simulink model "sm_tVtest_belt_IdlerArm_i2u0r3_underc"  (R2026a)
settings: Solver=VariableStepAuto  AbsTol=1e-3  EnableMultiTasking=on
undefined symbols (not defined in the file or in its folder): X, Y, Z
libraries: sm_lib x3, nesl_utility x1, sm_trackV_lib_belt_underc_idlerArm_i2u0l3 x1
Description:
  | Undercarriage with Frame and Rollers
  | Copyright 2024-2026 The MathWorks, Inc.
settings Model: Creator=smiller  LastModifiedBy=smiller
settings DebuggingCC: SubsystemReferenceDiagnosticForUnitTest=warning
settings SimscapeCC: SimscapeNominalValues="[{\"value\":\"1\",\"unit\":\"A\"},{\"value\":\"1\",\"unit\":\"bar\"},{\"value\":\"1\",\"unit\":\"cm^2\"},{\"value\":\"1\",\"unit\":\"cm^3/s\"},{\"value\":\"1\",\"unit\":\"kJ/kg\"},{\"value\":\"1\",\"unit\":\"kW\"},{\"value\":\"1\",\"unit\":\"l\"},{\"value\":\"1\",\"unit\":\"N\"},{\"value\":\"1\",\"unit\":\"N*m\"},{\"value\":\"1\",\"unit\":\"V\"}]"  SimscapeLogSimulationStatistics=on
settings DiagnosticsConfigSet: SimMechanicsUnconnectedFramePorts=none
settings ExplorerConfigSet: InternalSimMechanicsExplorerSettings="<ExplorerConfiguration><canonicalview>default</canonicalview><AnimationSetting><BasePlaybackSpeed>1.0</BasePlaybackSpeed><PlaybackSpeedFactor>1.0</PlaybackSpeedFactor></AnimationSetting><TilePanel><TileInfo><Tiles Columns=\"1\" Count=\"1\" Rows=\"1\"><Column Weight=\"1\"/><Row Weight=\"1\"/><Tile Height=\"1\" Width=\"1\" X=\"0\" Y=\"0\"/></Tiles></TileInfo><SceneInfo><SceneViewer><BGColor><R>1</R><G>1</G><B>1</B></BGColor><Camera><DoPerspective>off</DoPerspective><Position><X>0.903819359798529898</X><Y>-1.50805374329867981</Y><Z>-0.0280681494083976357</Z></Position><Center><X>-0.024120903320636794</X><Y>0.0864471732189572295</Y><Z>-0.450624958415139831</Z></Center><Up><X>-0.126434618294550744</X><Y>0.184704601083858</Y><Z>0.974627363475479402</Z></Up><ViewLimDist>1</ViewLimDist><YLim>1.06143678903579719</YLim><XLim>1.81016071934892686</XLim></Camera></SceneViewer></SceneInfo></TilePanel><MechEditorPanel><Cameras/><GfxPanelCameraMap/><VideoCreator><PlaybackSpeedRatio>1.0</PlaybackSpeedRatio><FrameRate>30</FrameRate><VideoFormat>Motion JPEG AVI</VideoFormat><FrameSize>auto</FrameSize></VideoCreator></MechEditorPanel></ExplorerConfiguration>"

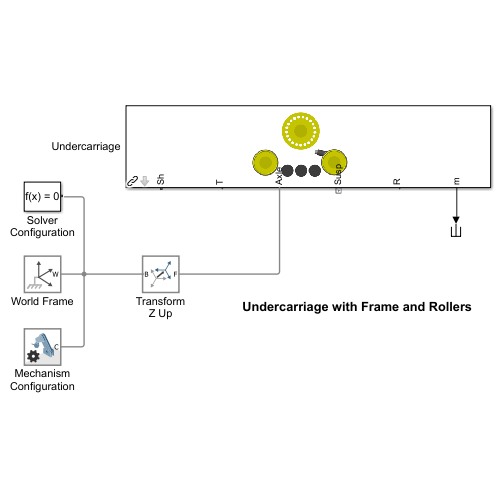
[thumbnail: Simulink's stored preview of the top-level diagram]
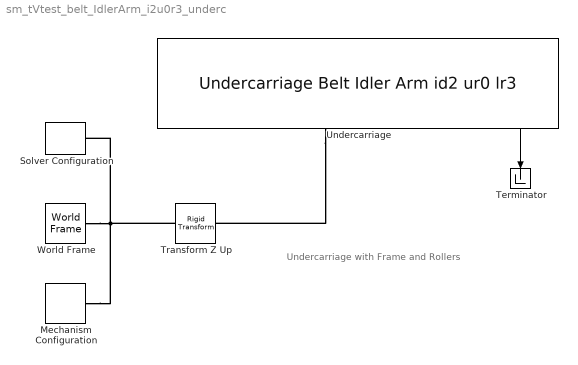
== system sm_tVtest_belt_IdlerArm_i2u0r3_underc ==
  note: Undercarriage with Frame and Rollers
  Mechanism Configuration : sm_lib/Utilities/Mechanism Configuration  UniformGravity=Constant  GravityVector=[0 0 -9.80665]  GravityVectorUnits=m/s^2  LinearizationDelta=0.001  JointModeTransitionNonlinearIterations=2
  Solver Configuration : nesl_utility/Solver Configuration  PhysicalDomain=network_engine_domain  SubClassName=solver  LeftPortType=input  RightPortType=generic  Tones=[]  Harmonics=[]  SimulateNoise=off  Profile=off  UseLocalSampling=off  EnableSwitchedLinearOptims=on  FrequencyDomain=off  UseCCode=off  RelTol=0.001  AbsTol=1e-06  MinStep=1e-09  ToWorkspace=off  RevertToSquareIcSolve=off  NumHomotopyIterations=100  PhasorMode=off  PhasorModeNumHarmonics=1  ConsistencySolver=NEWTON_XTOL_AFTER_FTOL  CanonicalOrdering=UNORDERED  OptimizeIntermediates=UNOPTIMIZED  IndexReductionMethod=DerivativeReplacement  DoDC=off  ResidualTolerance=1e-09  ConsistencyTolSource=GLOBAL  ConsistencyAbsTol=0.001  ConsistencyRelTol=0.001  ConsistencyTolFactor=0.001  UseLocalSolver=off  LocalSolverChoice=NE_BACKWARD_EULER_ADVANCER  ResolveIndetEquations=on  FunctionEvalNumThread=1  LocalSolverSampleTime=0.001  DoFixedCost=off  MaxNonlinIter=3  MaxModeIter=2  ComputeImpulses=off  ImpulseIterations=2  LinearAlgebra=Sparse  LinearAlgebraNumThread=0  EquationFormulation=NE_TIME_EF  DelaysMemoryBudget=1024  AutomaticFiltering=on  FilteringTimeConstant=0.001  PartitionStorageMethod=AS_NEEDED  PartitionMemoryBudget=1024  PartitionMethod=FAST  MultibodyUseLocalSolver=off  MultibodyLocalSolverChoice=ODE1  MultibodyLocalSolverSampleTime=0.001
  Terminator : Terminator
  Transform Z Up : sm_lib/Frames and Transforms/Rigid Transform  RotationMethod=StandardAxis  FollAlignAxisA=+X  BaseAlignAxisA=+Y  FollAlignAxisB=+Y  BaseAlignAxisB=+Z  RotationStandardAxis=+X  RotationAngle=-90  RotationAngleUnits=deg  RotationArbitraryAxis=[0 0 1]  RotationSequenceAxes=FollowerAxes  RotationSequence=XYX  RotationSequenceAngles=[0 0 0]  RotationSequenceAnglesUnits=deg  RotationMatrix=[1 0 0; 0 1 0; 0 0 1]  Quaternion=[1 0 0 0]  TranslationMethod=None  TranslationCartesianOffset=[0 0 0]  TranslationCartesianOffsetUnits=m  TranslationStandardAxis=+Z  TranslationStandardOffset=0  TranslationStandardOffsetUnits=m  TranslationROffset=0  TranslationROffsetUnits=m  TranslationThetaOffset=0  TranslationThetaOffsetUnits=deg  TranslationZOffset=0  TranslationZOffsetUnits=m
  Undercarriage : sm_trackV_lib_belt_underc_idlerArm_i2u0l3/Undercarriage Belt Idler Arm id2 ur0 lr3  popup_leftOrRight=Right  sprk_rad_roll=Trac.Sprocket.Roller.rad  sprk_wid_roll=Trac.Sprocket.Roller.wid  sprk_clr=Trac.Sprocket.Roller.clr  sprk_opc=Trac.Sprocket.Roller.opc  sprk_rim_ir=Trac.Sprocket.Rim.rad_inner  sprk_rim_thk=Trac.Sprocket.Rim.thk  sprk_rim_spoke_xc=Trac.Sprocket.Rim.spoke_xc  sprk_rad_pitch=Trac.Sprocket.Spoke.pitch_rad  sprk_spoke_rad=Trac.Sprocket.Spoke.rad  sprk_spoke_len=Trac.Sprocket.Spoke.len  sprk_spoke_num=Trac.Sprocket.nSpokes  sprk_contgeo_roller_clr=Trac.Sprocket.roller_contact.clr  sprk_contgeo_roller_opc=Trac.Sprocket.roller_contact.opc  sprk_contgeo_spoke_clr=Trac.Sprocket.spoke_contact.clr  sprk_contgeo_spoke_opc=Trac.Sprocket.spoke_contact.opc  idlerR_rad=Trac.IdlerR.rad  idlerF_rad=Trac.IdlerF.rad  idlerR_len=Trac.IdlerR.len  idlerF_len=Trac.IdlerF.len  idlerR_rho=Trac.IdlerR.rho  idlerF_rho=Trac.IdlerF.rho  idlerR_wheel_clr=Trac.IdlerR.Wheel.clr  idlerF_wheel_clr=Trac.IdlerF.Wheel.clr  idlerR_rim_rad=Trac.IdlerR.Rim.rad  idlerF_rim_rad=Trac.IdlerF.Rim.rad  idlerR_rim_hub_rad=Trac.IdlerR.Rim.hub_rad  idlerF_rim_hub_rad=Trac.IdlerF.Rim.hub_rad  idlerR_rim_xc=Trac.IdlerR.Rim.rim_xc  idlerF_rim_xc=Trac.IdlerF.Rim.rim_xc  idlerR_clr=Trac.IdlerR.clr  idlerF_clr=Trac.IdlerF.clr  idlerR_opc=Trac.IdlerR.opc  idlerF_opc=Trac.IdlerF.opc  idlerR_axle_rad=Trac.IdlerR.Axle.rad  idlerF_axle_rad=Trac.IdlerF.Axle.rad  idlerR_axle_len=Trac.IdlerR.Axle.len  idlerF_axle_len=Trac.IdlerF.Axle.len  idlerR_axle_rho=Trac.IdlerR.Axle.rho  idlerF_axle_rho=Trac.IdlerF.Axle.rho  idlerR_axle_clr=Trac.IdlerR.Axle.clr  idlerF_axle_clr=Trac.IdlerF.Axle.clr  idlerR_axle_opc=Trac.IdlerR.Axle.opc  idlerF_axle_opc=Trac.IdlerF.Axle.opc  idlerR_contgeo_clr=Trac.IdlerR.belt_contact.clr  idlerF_contgeo_clr=Trac.IdlerF.belt_contact.clr  idlerR_contgeo_opc=Trac.IdlerR.belt_contact.opc  idlerF_contgeo_opc=Trac.IdlerF.belt_contact.opc  arm_idlerc=Trac.IdlerArm.Pivot_to_Idler  arm_tens_x=Trac.IdlerArm.Pivot_to_TensionerX  arm_tens_y=Trac.IdlerArm.Pivot_to_TensionerY  arm_wid=Trac.IdlerArm.wid  arm_thk=Trac.IdlerArm.thk  arm_rho=Trac.IdlerArm.rho  arm_clr=Trac.IdlerArm.clr  arm_opc=Trac.IdlerArm.opc  roller_lower_len=Trac.Roller.Lower.len  roller_lower_rad=Trac.Roller.Lower.rad  roller_lower_rho=Trac.Roller.Lower.rho  roller_lower_clr=Trac.Roller.Lower.clr  roller_lower_opc=Trac.Roller.Lower.opc  roller_lower_rim_thk=Trac.Roller.Lower.rim_thk  roller_lower_rim_len=Trac.Roller.Lower.rim_len  roller_lower_axle_len=Trac.Roller.Lower.Axle.len  roller_lower_axle_rad=Trac.Roller.Lower.Axle.rad  roller_lower_axle_rho=Trac.Roller.Lower.Axle.rho  roller_lower_axle_clr=Trac.Roller.Lower.Axle.clr  roller_lower_axle_opc=Trac.Roller.Lower.Axle.opc  roller_lower_contgeo_clr=Trac.Roller.Lower.belt_contact.clr  roller_lower_contgeo_opc=Trac.Roller.Lower.belt_contact.opc  tensioner_cyl_len=Trac.IdlerF.Tensioner.cyl.len  tensioner_cyl_rad=Trac.IdlerF.Tensioner.cyl.rad  tensioner_cyl_rho=Trac.IdlerF.Tensioner.cyl.rho  tensioner_cyl_clr=Trac.IdlerF.Tensioner.cyl.clr  tensioner_cyl_opc=Trac.IdlerF.Tensioner.cyl.opc  tensioner_pist_len=Trac.IdlerF.Tensioner.piston.len  tensioner_pist_rad=Trac.IdlerF.Tensioner.piston.rad  tensioner_pist_rho=Trac.IdlerF.Tensioner.piston.rho  tensioner_pist_clr=Trac.IdlerF.Tensioner.piston.clr  tensioner_pist_opc=Trac.IdlerF.Tensioner.piston.opc  tensioner_br_len=Trac.IdlerF.Tensioner.bracket.len  tensioner_br_width=Trac.IdlerF.Tensioner.bracket.wid  tensioner_br_height=Trac.IdlerF.Tensioner.bracket.height  tensioner_br_thk=Trac.IdlerF.Tensioner.bracket.thk  tensioner_br_rho=Trac.IdlerF.Tensioner.bracket.rho  tensioner_br_clr=Trac.IdlerF.Tensioner.bracket.clr  tensioner_br_opc=Trac.IdlerF.Tensioner.bracket.opc  tensioner_eqpos=Trac.IdlerF.Tensioner.xeq  tensioner_x0=Trac.IdlerF.Tensioner.x0  tensioner_k=Trac.IdlerF.Tensioner.K  tensioner_b=Trac.IdlerF.Tensioner.B  popup_trackFrame=Fixed  roller_lower_x=Trac.Frame.SprkOffLon.Lower  axle_x=Trac.Frame.SprkOffLon.Axle  idlerFix_x=Trac.Frame.SprkOffLon.IdlerR  frame_pivot_x=Trac.Frame.SprkOffLon.PivotFra  tensionC_x=Trac.Frame.SprkOffLon.TensionC  idlerArm_x=Trac.Frame.SprkOffLon.IdlerArm  roller_lower_y=Trac.Frame.SprkOffVer.Lower  axle_y=Trac.Frame.SprkOffVer.Axle  idlerArm_y=Trac.Frame.SprkOffVer.IdlerArm  idlerFix_y=Trac.Frame.SprkOffVer.IdlerR  frame_pivot_y=Trac.Frame.SprkOffVer.PivotFra  tensionC_y=Trac.Frame.SprkOffVer.TensionC  frame_cg_offset=Trac.Frame.TrackFrame.CG  frame_mass=Trac.Frame.TrackFrame.Mass  frame_moi=Trac.Frame.TrackFrame.MOI  frame_poi=Trac.Frame.TrackFrame.POI  frame_roller_cg_offset=Trac.Frame.SprkFrame.CG  frame_roller_mass=Trac.Frame.SprkFrame.Mass  frame_roller_moi=Trac.Frame.SprkFrame.MOI  frame_roller_poi=Trac.Frame.SprkFrame.POI  roller_frame_pivot_range=Trac.Frame.PivotFra.Range  roller_frame_pivot_k=Trac.Frame.PivotFra.LimitK  roller_frame_pivot_b=Trac.Frame.PivotFra.LimitB  roller_frame_pivot_tw=Trac.Frame.PivotFra.LimitTW  frame_susp_offset=Trac.Frame.SuspOffset  popup_sense_roller=Actuator Torque
  World Frame : sm_lib/Frames and Transforms/World Frame
  wires:
  Undercarriage/1 -> Terminator/1
  connections:
  World Frame/RConn1 -- Transform Z Up/LConn1 -- Solver Configuration/RConn1 -- Mechanism Configuration/RConn1
  Undercarriage/RConn3 -- Transform Z Up/RConn1
